simulink model "TST_CrCtl_ShOff"  (R2016b)
settings: Solver=FixedStepDiscrete  StartTime=0.0  StopTime=simTime  FixedStep=sampleTime  RelTol=1e-3
values from neighbouring files (symbols this model uses):
  testCase = 1    [initTST_CrCtl_ShOff_001.m]    (also in initTST_CrCtl_ShOff_002.m = 2; initTST_CrCtl_ShOff_003.m = 3)
libraries: simulink x31, UnitTest_Lib x15
(part 2 of 2)

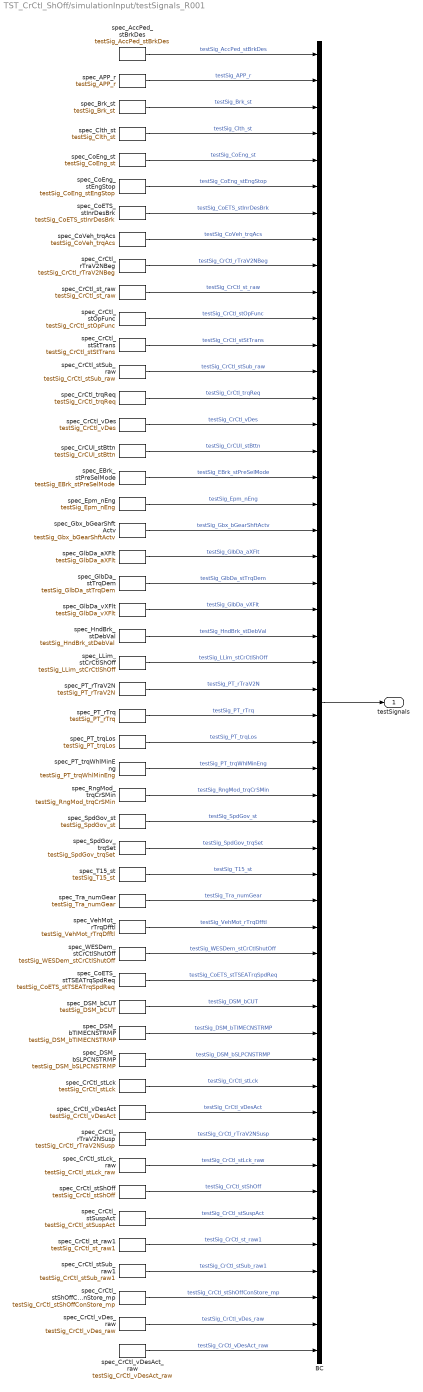
== system TST_CrCtl_ShOff/simulationInput/testSignals_R001 ==
  BC : BusCreator  Inputs=50
  spec_APP_r : FromWorkspace  VariableName=testSig_APP_r  Interpolate=off  OutputAfterFinalValue=Holding final value
  spec_AccPed_stBrkDes : FromWorkspace  VariableName=testSig_AccPed_stBrkDes  Interpolate=off  OutputAfterFinalValue=Holding final value
  spec_Brk_st : FromWorkspace  VariableName=testSig_Brk_st  Interpolate=off  OutputAfterFinalValue=Holding final value
  spec_Clth_st : FromWorkspace  VariableName=testSig_Clth_st  Interpolate=off  OutputAfterFinalValue=Holding final value
  spec_CoETS_stInrDesBrk : FromWorkspace  VariableName=testSig_CoETS_stInrDesBrk  Interpolate=off  OutputAfterFinalValue=Holding final value
  spec_CoETS_stTSEATrqSpdReq : FromWorkspace  VariableName=testSig_CoETS_stTSEATrqSpdReq  Interpolate=off  OutputAfterFinalValue=Holding final value
  spec_CoEng_st : FromWorkspace  VariableName=testSig_CoEng_st  Interpolate=off  OutputAfterFinalValue=Holding final value
  spec_CoEng_stEngStop : FromWorkspace  VariableName=testSig_CoEng_stEngStop  Interpolate=off  OutputAfterFinalValue=Holding final value
  spec_CoVeh_trqAcs : FromWorkspace  VariableName=testSig_CoVeh_trqAcs  Interpolate=off  OutputAfterFinalValue=Holding final value
  spec_CrCUI_stBttn : FromWorkspace  VariableName=testSig_CrCUI_stBttn  Interpolate=off  OutputAfterFinalValue=Holding final value
  spec_CrCtl_rTraV2NBeg : FromWorkspace  VariableName=testSig_CrCtl_rTraV2NBeg  Interpolate=off  OutputAfterFinalValue=Holding final value
  spec_CrCtl_rTraV2NSusp : FromWorkspace  VariableName=testSig_CrCtl_rTraV2NSusp  Interpolate=off  OutputAfterFinalValue=Holding final value
  spec_CrCtl_stLck : FromWorkspace  VariableName=testSig_CrCtl_stLck  Interpolate=off  OutputAfterFinalValue=Holding final value
  spec_CrCtl_stLck_raw : FromWorkspace  VariableName=testSig_CrCtl_stLck_raw  Interpolate=off  OutputAfterFinalValue=Holding final value
  spec_CrCtl_stOpFunc : FromWorkspace  VariableName=testSig_CrCtl_stOpFunc  Interpolate=off  OutputAfterFinalValue=Holding final value
  spec_CrCtl_stShOff : FromWorkspace  VariableName=testSig_CrCtl_stShOff  Interpolate=off  OutputAfterFinalValue=Holding final value
  spec_CrCtl_stShOffConStore_mp : FromWorkspace  VariableName=testSig_CrCtl_stShOffConStore_mp  Interpolate=off  OutputAfterFinalValue=Holding final value
  spec_CrCtl_stStTrans : FromWorkspace  VariableName=testSig_CrCtl_stStTrans  Interpolate=off  OutputAfterFinalValue=Holding final value
  spec_CrCtl_stSub_raw : FromWorkspace  VariableName=testSig_CrCtl_stSub_raw  Interpolate=off  OutputAfterFinalValue=Holding final value
  spec_CrCtl_stSub_raw1 : FromWorkspace  VariableName=testSig_CrCtl_stSub_raw1  Interpolate=off  OutputAfterFinalValue=Holding final value
  spec_CrCtl_stSuspAct : FromWorkspace  VariableName=testSig_CrCtl_stSuspAct  Interpolate=off  OutputAfterFinalValue=Holding final value
  spec_CrCtl_st_raw : FromWorkspace  VariableName=testSig_CrCtl_st_raw  Interpolate=off  OutputAfterFinalValue=Holding final value
  spec_CrCtl_st_raw1 : FromWorkspace  VariableName=testSig_CrCtl_st_raw1  Interpolate=off  OutputAfterFinalValue=Holding final value
  spec_CrCtl_trqReq : FromWorkspace  VariableName=testSig_CrCtl_trqReq  Interpolate=off  OutputAfterFinalValue=Holding final value
  spec_CrCtl_vDes : FromWorkspace  VariableName=testSig_CrCtl_vDes  Interpolate=off  OutputAfterFinalValue=Holding final value
  spec_CrCtl_vDesAct : FromWorkspace  VariableName=testSig_CrCtl_vDesAct  Interpolate=off  OutputAfterFinalValue=Holding final value
  spec_CrCtl_vDesAct_raw : FromWorkspace  VariableName=testSig_CrCtl_vDesAct_raw  Interpolate=off  OutputAfterFinalValue=Holding final value
  spec_CrCtl_vDes_raw : FromWorkspace  VariableName=testSig_CrCtl_vDes_raw  Interpolate=off  OutputAfterFinalValue=Holding final value
  spec_DSM_bCUT : FromWorkspace  VariableName=testSig_DSM_bCUT  Interpolate=off  OutputAfterFinalValue=Holding final value
  spec_DSM_bSLPCNSTRMP : FromWorkspace  VariableName=testSig_DSM_bSLPCNSTRMP  Interpolate=off  OutputAfterFinalValue=Holding final value
  spec_DSM_bTIMECNSTRMP : FromWorkspace  VariableName=testSig_DSM_bTIMECNSTRMP  Interpolate=off  OutputAfterFinalValue=Holding final value
  spec_EBrk_stPreSelMode : FromWorkspace  VariableName=testSig_EBrk_stPreSelMode  Interpolate=off  OutputAfterFinalValue=Holding final value
  spec_Epm_nEng : FromWorkspace  VariableName=testSig_Epm_nEng  Interpolate=off  OutputAfterFinalValue=Holding final value
  spec_Gbx_bGearShftActv : FromWorkspace  VariableName=testSig_Gbx_bGearShftActv  Interpolate=off  OutputAfterFinalValue=Holding final value
  spec_GlbDa_aXFlt : FromWorkspace  VariableName=testSig_GlbDa_aXFlt  Interpolate=off  OutputAfterFinalValue=Holding final value
  spec_GlbDa_stTrqDem : FromWorkspace  VariableName=testSig_GlbDa_stTrqDem  Interpolate=off  OutputAfterFinalValue=Holding final value
  spec_GlbDa_vXFlt : FromWorkspace  VariableName=testSig_GlbDa_vXFlt  Interpolate=off  OutputAfterFinalValue=Holding final value
  spec_HndBrk_stDebVal : FromWorkspace  VariableName=testSig_HndBrk_stDebVal  Interpolate=off  OutputAfterFinalValue=Holding final value
  spec_LLim_stCrCtlShOff : FromWorkspace  VariableName=testSig_LLim_stCrCtlShOff  Interpolate=off  OutputAfterFinalValue=Holding final value
  spec_PT_rTraV2N : FromWorkspace  VariableName=testSig_PT_rTraV2N  Interpolate=off  OutputAfterFinalValue=Holding final value
  spec_PT_rTrq : FromWorkspace  VariableName=testSig_PT_rTrq  Interpolate=off  OutputAfterFinalValue=Holding final value
  spec_PT_trqLos : FromWorkspace  VariableName=testSig_PT_trqLos  Interpolate=off  OutputAfterFinalValue=Holding final value
  spec_PT_trqWhlMinEng : FromWorkspace  VariableName=testSig_PT_trqWhlMinEng  Interpolate=off  OutputAfterFinalValue=Holding final value
  spec_RngMod_trqCrSMin : FromWorkspace  VariableName=testSig_RngMod_trqCrSMin  Interpolate=off  OutputAfterFinalValue=Holding final value
  spec_SpdGov_st : FromWorkspace  VariableName=testSig_SpdGov_st  Interpolate=off  OutputAfterFinalValue=Holding final value
  spec_SpdGov_trqSet : FromWorkspace  VariableName=testSig_SpdGov_trqSet  Interpolate=off  OutputAfterFinalValue=Holding final value
  spec_T15_st : FromWorkspace  VariableName=testSig_T15_st  Interpolate=off  OutputAfterFinalValue=Holding final value
  spec_Tra_numGear : FromWorkspace  VariableName=testSig_Tra_numGear  Interpolate=off  OutputAfterFinalValue=Holding final value
  spec_VehMot_rTrqDfftl : FromWorkspace  VariableName=testSig_VehMot_rTrqDfftl  Interpolate=off  OutputAfterFinalValue=Holding final value
  spec_WESDem_stCrCtlShutOff : FromWorkspace  VariableName=testSig_WESDem_stCrCtlShutOff  Interpolate=off  OutputAfterFinalValue=Holding final value
  testSignals : Outport
  wires:
  BC/1 -> testSignals/1
  spec_AccPed_stBrkDes/1 -> BC/1  "testSig_AccPed_stBrkDes"
  spec_APP_r/1 -> BC/2  "testSig_APP_r"
  spec_Brk_st/1 -> BC/3  "testSig_Brk_st"
  spec_Clth_st/1 -> BC/4  "testSig_Clth_st"
  spec_CoEng_st/1 -> BC/5  "testSig_CoEng_st"
  spec_CoEng_stEngStop/1 -> BC/6  "testSig_CoEng_stEngStop"
  spec_CoETS_stInrDesBrk/1 -> BC/7  "testSig_CoETS_stInrDesBrk"
  spec_CoVeh_trqAcs/1 -> BC/8  "testSig_CoVeh_trqAcs"
  spec_CrCtl_rTraV2NBeg/1 -> BC/9  "testSig_CrCtl_rTraV2NBeg"
  spec_CrCtl_st_raw/1 -> BC/10  "testSig_CrCtl_st_raw"
  spec_CrCtl_stOpFunc/1 -> BC/11  "testSig_CrCtl_stOpFunc"
  spec_CrCtl_stStTrans/1 -> BC/12  "testSig_CrCtl_stStTrans"
  spec_CrCtl_stSub_raw/1 -> BC/13  "testSig_CrCtl_stSub_raw"
  spec_CrCtl_trqReq/1 -> BC/14  "testSig_CrCtl_trqReq"
  spec_CrCtl_vDes/1 -> BC/15  "testSig_CrCtl_vDes"
  spec_CrCUI_stBttn/1 -> BC/16  "testSig_CrCUI_stBttn"
  spec_EBrk_stPreSelMode/1 -> BC/17  "testSig_EBrk_stPreSelMode"
  spec_Epm_nEng/1 -> BC/18  "testSig_Epm_nEng"
  spec_Gbx_bGearShftActv/1 -> BC/19  "testSig_Gbx_bGearShftActv"
  spec_GlbDa_aXFlt/1 -> BC/20  "testSig_GlbDa_aXFlt"
  spec_GlbDa_stTrqDem/1 -> BC/21  "testSig_GlbDa_stTrqDem"
  spec_GlbDa_vXFlt/1 -> BC/22  "testSig_GlbDa_vXFlt"
  spec_HndBrk_stDebVal/1 -> BC/23  "testSig_HndBrk_stDebVal"
  spec_LLim_stCrCtlShOff/1 -> BC/24  "testSig_LLim_stCrCtlShOff"
  spec_PT_rTraV2N/1 -> BC/25  "testSig_PT_rTraV2N"
  spec_PT_rTrq/1 -> BC/26  "testSig_PT_rTrq"
  spec_PT_trqLos/1 -> BC/27  "testSig_PT_trqLos"
  spec_PT_trqWhlMinEng/1 -> BC/28  "testSig_PT_trqWhlMinEng"
  spec_RngMod_trqCrSMin/1 -> BC/29  "testSig_RngMod_trqCrSMin"
  spec_SpdGov_st/1 -> BC/30  "testSig_SpdGov_st"
  spec_SpdGov_trqSet/1 -> BC/31  "testSig_SpdGov_trqSet"
  spec_T15_st/1 -> BC/32  "testSig_T15_st"
  spec_Tra_numGear/1 -> BC/33  "testSig_Tra_numGear"
  spec_VehMot_rTrqDfftl/1 -> BC/34  "testSig_VehMot_rTrqDfftl"
  spec_WESDem_stCrCtlShutOff/1 -> BC/35  "testSig_WESDem_stCrCtlShutOff"
  spec_CoETS_stTSEATrqSpdReq/1 -> BC/36  "testSig_CoETS_stTSEATrqSpdReq"
  spec_DSM_bCUT/1 -> BC/37  "testSig_DSM_bCUT"
  spec_DSM_bTIMECNSTRMP/1 -> BC/38  "testSig_DSM_bTIMECNSTRMP"
  spec_DSM_bSLPCNSTRMP/1 -> BC/39  "testSig_DSM_bSLPCNSTRMP"
  spec_CrCtl_stLck/1 -> BC/40  "testSig_CrCtl_stLck"
  spec_CrCtl_vDesAct/1 -> BC/41  "testSig_CrCtl_vDesAct"
  spec_CrCtl_rTraV2NSusp/1 -> BC/42  "testSig_CrCtl_rTraV2NSusp"
  spec_CrCtl_stLck_raw/1 -> BC/43  "testSig_CrCtl_stLck_raw"
  spec_CrCtl_stShOff/1 -> BC/44  "testSig_CrCtl_stShOff"
  spec_CrCtl_stSuspAct/1 -> BC/45  "testSig_CrCtl_stSuspAct"
  spec_CrCtl_st_raw1/1 -> BC/46  "testSig_CrCtl_st_raw1"
  spec_CrCtl_stSub_raw1/1 -> BC/47  "testSig_CrCtl_stSub_raw1"
  spec_CrCtl_stShOffConStore_mp/1 -> BC/48  "testSig_CrCtl_stShOffConStore_mp"
  spec_CrCtl_vDes_raw/1 -> BC/49  "testSig_CrCtl_vDes_raw"
  spec_CrCtl_vDesAct_raw/1 -> BC/50  "testSig_CrCtl_vDesAct_raw"

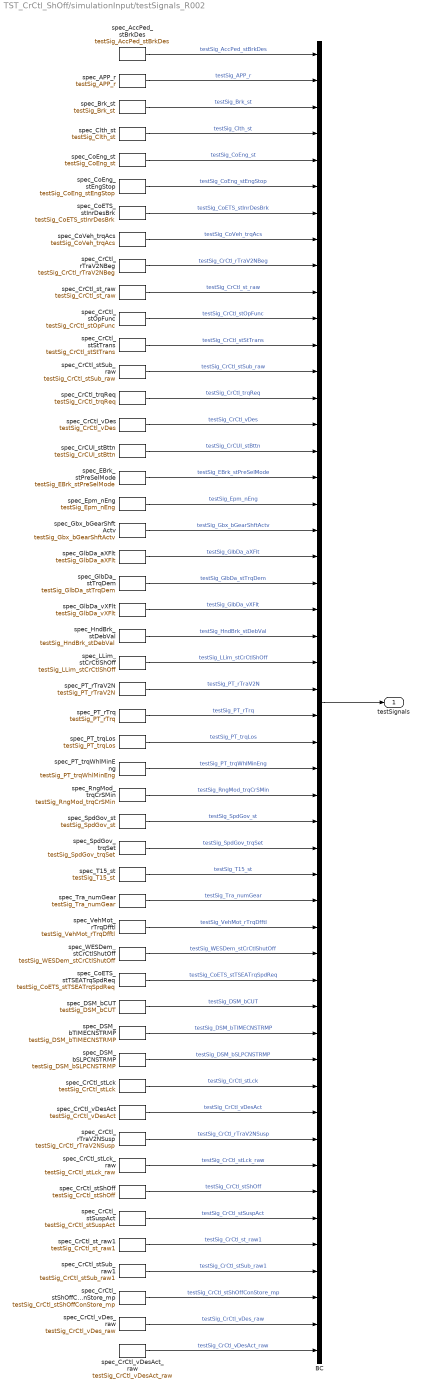
== system TST_CrCtl_ShOff/simulationInput/testSignals_R002 ==
  BC : BusCreator  Inputs=50
  spec_APP_r : FromWorkspace  VariableName=testSig_APP_r  Interpolate=off  OutputAfterFinalValue=Holding final value
  spec_AccPed_stBrkDes : FromWorkspace  VariableName=testSig_AccPed_stBrkDes  Interpolate=off  OutputAfterFinalValue=Holding final value
  spec_Brk_st : FromWorkspace  VariableName=testSig_Brk_st  Interpolate=off  OutputAfterFinalValue=Holding final value
  spec_Clth_st : FromWorkspace  VariableName=testSig_Clth_st  Interpolate=off  OutputAfterFinalValue=Holding final value
  spec_CoETS_stInrDesBrk : FromWorkspace  VariableName=testSig_CoETS_stInrDesBrk  Interpolate=off  OutputAfterFinalValue=Holding final value
  spec_CoETS_stTSEATrqSpdReq : FromWorkspace  VariableName=testSig_CoETS_stTSEATrqSpdReq  Interpolate=off  OutputAfterFinalValue=Holding final value
  spec_CoEng_st : FromWorkspace  VariableName=testSig_CoEng_st  Interpolate=off  OutputAfterFinalValue=Holding final value
  spec_CoEng_stEngStop : FromWorkspace  VariableName=testSig_CoEng_stEngStop  Interpolate=off  OutputAfterFinalValue=Holding final value
  spec_CoVeh_trqAcs : FromWorkspace  VariableName=testSig_CoVeh_trqAcs  Interpolate=off  OutputAfterFinalValue=Holding final value
  spec_CrCUI_stBttn : FromWorkspace  VariableName=testSig_CrCUI_stBttn  Interpolate=off  OutputAfterFinalValue=Holding final value
  spec_CrCtl_rTraV2NBeg : FromWorkspace  VariableName=testSig_CrCtl_rTraV2NBeg  Interpolate=off  OutputAfterFinalValue=Holding final value
  spec_CrCtl_rTraV2NSusp : FromWorkspace  VariableName=testSig_CrCtl_rTraV2NSusp  Interpolate=off  OutputAfterFinalValue=Holding final value
  spec_CrCtl_stLck : FromWorkspace  VariableName=testSig_CrCtl_stLck  Interpolate=off  OutputAfterFinalValue=Holding final value
  spec_CrCtl_stLck_raw : FromWorkspace  VariableName=testSig_CrCtl_stLck_raw  Interpolate=off  OutputAfterFinalValue=Holding final value
  spec_CrCtl_stOpFunc : FromWorkspace  VariableName=testSig_CrCtl_stOpFunc  Interpolate=off  OutputAfterFinalValue=Holding final value
  spec_CrCtl_stShOff : FromWorkspace  VariableName=testSig_CrCtl_stShOff  Interpolate=off  OutputAfterFinalValue=Holding final value
  spec_CrCtl_stShOffConStore_mp : FromWorkspace  VariableName=testSig_CrCtl_stShOffConStore_mp  Interpolate=off  OutputAfterFinalValue=Holding final value
  spec_CrCtl_stStTrans : FromWorkspace  VariableName=testSig_CrCtl_stStTrans  Interpolate=off  OutputAfterFinalValue=Holding final value
  spec_CrCtl_stSub_raw : FromWorkspace  VariableName=testSig_CrCtl_stSub_raw  Interpolate=off  OutputAfterFinalValue=Holding final value
  spec_CrCtl_stSub_raw1 : FromWorkspace  VariableName=testSig_CrCtl_stSub_raw1  Interpolate=off  OutputAfterFinalValue=Holding final value
  spec_CrCtl_stSuspAct : FromWorkspace  VariableName=testSig_CrCtl_stSuspAct  Interpolate=off  OutputAfterFinalValue=Holding final value
  spec_CrCtl_st_raw : FromWorkspace  VariableName=testSig_CrCtl_st_raw  Interpolate=off  OutputAfterFinalValue=Holding final value
  spec_CrCtl_st_raw1 : FromWorkspace  VariableName=testSig_CrCtl_st_raw1  Interpolate=off  OutputAfterFinalValue=Holding final value
  spec_CrCtl_trqReq : FromWorkspace  VariableName=testSig_CrCtl_trqReq  Interpolate=off  OutputAfterFinalValue=Holding final value
  spec_CrCtl_vDes : FromWorkspace  VariableName=testSig_CrCtl_vDes  Interpolate=off  OutputAfterFinalValue=Holding final value
  spec_CrCtl_vDesAct : FromWorkspace  VariableName=testSig_CrCtl_vDesAct  Interpolate=off  OutputAfterFinalValue=Holding final value
  spec_CrCtl_vDesAct_raw : FromWorkspace  VariableName=testSig_CrCtl_vDesAct_raw  Interpolate=off  OutputAfterFinalValue=Holding final value
  spec_CrCtl_vDes_raw : FromWorkspace  VariableName=testSig_CrCtl_vDes_raw  Interpolate=off  OutputAfterFinalValue=Holding final value
  spec_DSM_bCUT : FromWorkspace  VariableName=testSig_DSM_bCUT  Interpolate=off  OutputAfterFinalValue=Holding final value
  spec_DSM_bSLPCNSTRMP : FromWorkspace  VariableName=testSig_DSM_bSLPCNSTRMP  Interpolate=off  OutputAfterFinalValue=Holding final value
  spec_DSM_bTIMECNSTRMP : FromWorkspace  VariableName=testSig_DSM_bTIMECNSTRMP  Interpolate=off  OutputAfterFinalValue=Holding final value
  spec_EBrk_stPreSelMode : FromWorkspace  VariableName=testSig_EBrk_stPreSelMode  Interpolate=off  OutputAfterFinalValue=Holding final value
  spec_Epm_nEng : FromWorkspace  VariableName=testSig_Epm_nEng  Interpolate=off  OutputAfterFinalValue=Holding final value
  spec_Gbx_bGearShftActv : FromWorkspace  VariableName=testSig_Gbx_bGearShftActv  Interpolate=off  OutputAfterFinalValue=Holding final value
  spec_GlbDa_aXFlt : FromWorkspace  VariableName=testSig_GlbDa_aXFlt  Interpolate=off  OutputAfterFinalValue=Holding final value
  spec_GlbDa_stTrqDem : FromWorkspace  VariableName=testSig_GlbDa_stTrqDem  Interpolate=off  OutputAfterFinalValue=Holding final value
  spec_GlbDa_vXFlt : FromWorkspace  VariableName=testSig_GlbDa_vXFlt  Interpolate=off  OutputAfterFinalValue=Holding final value
  spec_HndBrk_stDebVal : FromWorkspace  VariableName=testSig_HndBrk_stDebVal  Interpolate=off  OutputAfterFinalValue=Holding final value
  spec_LLim_stCrCtlShOff : FromWorkspace  VariableName=testSig_LLim_stCrCtlShOff  Interpolate=off  OutputAfterFinalValue=Holding final value
  spec_PT_rTraV2N : FromWorkspace  VariableName=testSig_PT_rTraV2N  Interpolate=off  OutputAfterFinalValue=Holding final value
  spec_PT_rTrq : FromWorkspace  VariableName=testSig_PT_rTrq  Interpolate=off  OutputAfterFinalValue=Holding final value
  spec_PT_trqLos : FromWorkspace  VariableName=testSig_PT_trqLos  Interpolate=off  OutputAfterFinalValue=Holding final value
  spec_PT_trqWhlMinEng : FromWorkspace  VariableName=testSig_PT_trqWhlMinEng  Interpolate=off  OutputAfterFinalValue=Holding final value
  spec_RngMod_trqCrSMin : FromWorkspace  VariableName=testSig_RngMod_trqCrSMin  Interpolate=off  OutputAfterFinalValue=Holding final value
  spec_SpdGov_st : FromWorkspace  VariableName=testSig_SpdGov_st  Interpolate=off  OutputAfterFinalValue=Holding final value
  spec_SpdGov_trqSet : FromWorkspace  VariableName=testSig_SpdGov_trqSet  Interpolate=off  OutputAfterFinalValue=Holding final value
  spec_T15_st : FromWorkspace  VariableName=testSig_T15_st  Interpolate=off  OutputAfterFinalValue=Holding final value
  spec_Tra_numGear : FromWorkspace  VariableName=testSig_Tra_numGear  Interpolate=off  OutputAfterFinalValue=Holding final value
  spec_VehMot_rTrqDfftl : FromWorkspace  VariableName=testSig_VehMot_rTrqDfftl  Interpolate=off  OutputAfterFinalValue=Holding final value
  spec_WESDem_stCrCtlShutOff : FromWorkspace  VariableName=testSig_WESDem_stCrCtlShutOff  Interpolate=off  OutputAfterFinalValue=Holding final value
  testSignals : Outport
  wires:
  BC/1 -> testSignals/1
  spec_AccPed_stBrkDes/1 -> BC/1  "testSig_AccPed_stBrkDes"
  spec_APP_r/1 -> BC/2  "testSig_APP_r"
  spec_Brk_st/1 -> BC/3  "testSig_Brk_st"
  spec_Clth_st/1 -> BC/4  "testSig_Clth_st"
  spec_CoEng_st/1 -> BC/5  "testSig_CoEng_st"
  spec_CoEng_stEngStop/1 -> BC/6  "testSig_CoEng_stEngStop"
  spec_CoETS_stInrDesBrk/1 -> BC/7  "testSig_CoETS_stInrDesBrk"
  spec_CoVeh_trqAcs/1 -> BC/8  "testSig_CoVeh_trqAcs"
  spec_CrCtl_rTraV2NBeg/1 -> BC/9  "testSig_CrCtl_rTraV2NBeg"
  spec_CrCtl_st_raw/1 -> BC/10  "testSig_CrCtl_st_raw"
  spec_CrCtl_stOpFunc/1 -> BC/11  "testSig_CrCtl_stOpFunc"
  spec_CrCtl_stStTrans/1 -> BC/12  "testSig_CrCtl_stStTrans"
  spec_CrCtl_stSub_raw/1 -> BC/13  "testSig_CrCtl_stSub_raw"
  spec_CrCtl_trqReq/1 -> BC/14  "testSig_CrCtl_trqReq"
  spec_CrCtl_vDes/1 -> BC/15  "testSig_CrCtl_vDes"
  spec_CrCUI_stBttn/1 -> BC/16  "testSig_CrCUI_stBttn"
  spec_EBrk_stPreSelMode/1 -> BC/17  "testSig_EBrk_stPreSelMode"
  spec_Epm_nEng/1 -> BC/18  "testSig_Epm_nEng"
  spec_Gbx_bGearShftActv/1 -> BC/19  "testSig_Gbx_bGearShftActv"
  spec_GlbDa_aXFlt/1 -> BC/20  "testSig_GlbDa_aXFlt"
  spec_GlbDa_stTrqDem/1 -> BC/21  "testSig_GlbDa_stTrqDem"
  spec_GlbDa_vXFlt/1 -> BC/22  "testSig_GlbDa_vXFlt"
  spec_HndBrk_stDebVal/1 -> BC/23  "testSig_HndBrk_stDebVal"
  spec_LLim_stCrCtlShOff/1 -> BC/24  "testSig_LLim_stCrCtlShOff"
  spec_PT_rTraV2N/1 -> BC/25  "testSig_PT_rTraV2N"
  spec_PT_rTrq/1 -> BC/26  "testSig_PT_rTrq"
  spec_PT_trqLos/1 -> BC/27  "testSig_PT_trqLos"
  spec_PT_trqWhlMinEng/1 -> BC/28  "testSig_PT_trqWhlMinEng"
  spec_RngMod_trqCrSMin/1 -> BC/29  "testSig_RngMod_trqCrSMin"
  spec_SpdGov_st/1 -> BC/30  "testSig_SpdGov_st"
  spec_SpdGov_trqSet/1 -> BC/31  "testSig_SpdGov_trqSet"
  spec_T15_st/1 -> BC/32  "testSig_T15_st"
  spec_Tra_numGear/1 -> BC/33  "testSig_Tra_numGear"
  spec_VehMot_rTrqDfftl/1 -> BC/34  "testSig_VehMot_rTrqDfftl"
  spec_WESDem_stCrCtlShutOff/1 -> BC/35  "testSig_WESDem_stCrCtlShutOff"
  spec_CoETS_stTSEATrqSpdReq/1 -> BC/36  "testSig_CoETS_stTSEATrqSpdReq"
  spec_DSM_bCUT/1 -> BC/37  "testSig_DSM_bCUT"
  spec_DSM_bTIMECNSTRMP/1 -> BC/38  "testSig_DSM_bTIMECNSTRMP"
  spec_DSM_bSLPCNSTRMP/1 -> BC/39  "testSig_DSM_bSLPCNSTRMP"
  spec_CrCtl_stLck/1 -> BC/40  "testSig_CrCtl_stLck"
  spec_CrCtl_vDesAct/1 -> BC/41  "testSig_CrCtl_vDesAct"
  spec_CrCtl_rTraV2NSusp/1 -> BC/42  "testSig_CrCtl_rTraV2NSusp"
  spec_CrCtl_stLck_raw/1 -> BC/43  "testSig_CrCtl_stLck_raw"
  spec_CrCtl_stShOff/1 -> BC/44  "testSig_CrCtl_stShOff"
  spec_CrCtl_stSuspAct/1 -> BC/45  "testSig_CrCtl_stSuspAct"
  spec_CrCtl_st_raw1/1 -> BC/46  "testSig_CrCtl_st_raw1"
  spec_CrCtl_stSub_raw1/1 -> BC/47  "testSig_CrCtl_stSub_raw1"
  spec_CrCtl_stShOffConStore_mp/1 -> BC/48  "testSig_CrCtl_stShOffConStore_mp"
  spec_CrCtl_vDes_raw/1 -> BC/49  "testSig_CrCtl_vDes_raw"
  spec_CrCtl_vDesAct_raw/1 -> BC/50  "testSig_CrCtl_vDesAct_raw"

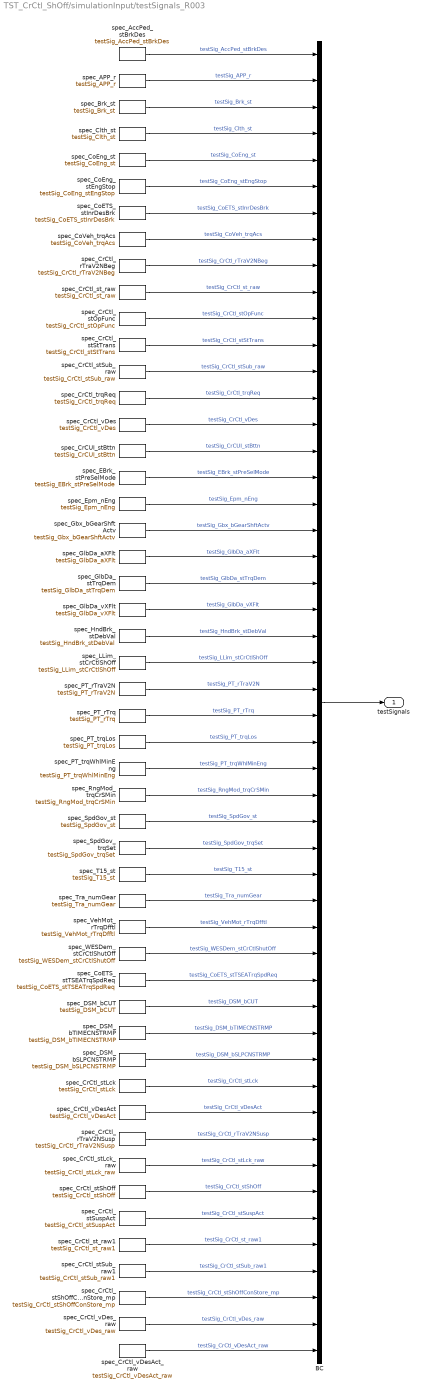
== system TST_CrCtl_ShOff/simulationInput/testSignals_R003 ==
  BC : BusCreator  Inputs=50
  spec_APP_r : FromWorkspace  VariableName=testSig_APP_r  Interpolate=off  OutputAfterFinalValue=Holding final value
  spec_AccPed_stBrkDes : FromWorkspace  VariableName=testSig_AccPed_stBrkDes  Interpolate=off  OutputAfterFinalValue=Holding final value
  spec_Brk_st : FromWorkspace  VariableName=testSig_Brk_st  Interpolate=off  OutputAfterFinalValue=Holding final value
  spec_Clth_st : FromWorkspace  VariableName=testSig_Clth_st  Interpolate=off  OutputAfterFinalValue=Holding final value
  spec_CoETS_stInrDesBrk : FromWorkspace  VariableName=testSig_CoETS_stInrDesBrk  Interpolate=off  OutputAfterFinalValue=Holding final value
  spec_CoETS_stTSEATrqSpdReq : FromWorkspace  VariableName=testSig_CoETS_stTSEATrqSpdReq  Interpolate=off  OutputAfterFinalValue=Holding final value
  spec_CoEng_st : FromWorkspace  VariableName=testSig_CoEng_st  Interpolate=off  OutputAfterFinalValue=Holding final value
  spec_CoEng_stEngStop : FromWorkspace  VariableName=testSig_CoEng_stEngStop  Interpolate=off  OutputAfterFinalValue=Holding final value
  spec_CoVeh_trqAcs : FromWorkspace  VariableName=testSig_CoVeh_trqAcs  Interpolate=off  OutputAfterFinalValue=Holding final value
  spec_CrCUI_stBttn : FromWorkspace  VariableName=testSig_CrCUI_stBttn  Interpolate=off  OutputAfterFinalValue=Holding final value
  spec_CrCtl_rTraV2NBeg : FromWorkspace  VariableName=testSig_CrCtl_rTraV2NBeg  Interpolate=off  OutputAfterFinalValue=Holding final value
  spec_CrCtl_rTraV2NSusp : FromWorkspace  VariableName=testSig_CrCtl_rTraV2NSusp  Interpolate=off  OutputAfterFinalValue=Holding final value
  spec_CrCtl_stLck : FromWorkspace  VariableName=testSig_CrCtl_stLck  Interpolate=off  OutputAfterFinalValue=Holding final value
  spec_CrCtl_stLck_raw : FromWorkspace  VariableName=testSig_CrCtl_stLck_raw  Interpolate=off  OutputAfterFinalValue=Holding final value
  spec_CrCtl_stOpFunc : FromWorkspace  VariableName=testSig_CrCtl_stOpFunc  Interpolate=off  OutputAfterFinalValue=Holding final value
  spec_CrCtl_stShOff : FromWorkspace  VariableName=testSig_CrCtl_stShOff  Interpolate=off  OutputAfterFinalValue=Holding final value
  spec_CrCtl_stShOffConStore_mp : FromWorkspace  VariableName=testSig_CrCtl_stShOffConStore_mp  Interpolate=off  OutputAfterFinalValue=Holding final value
  spec_CrCtl_stStTrans : FromWorkspace  VariableName=testSig_CrCtl_stStTrans  Interpolate=off  OutputAfterFinalValue=Holding final value
  spec_CrCtl_stSub_raw : FromWorkspace  VariableName=testSig_CrCtl_stSub_raw  Interpolate=off  OutputAfterFinalValue=Holding final value
  spec_CrCtl_stSub_raw1 : FromWorkspace  VariableName=testSig_CrCtl_stSub_raw1  Interpolate=off  OutputAfterFinalValue=Holding final value
  spec_CrCtl_stSuspAct : FromWorkspace  VariableName=testSig_CrCtl_stSuspAct  Interpolate=off  OutputAfterFinalValue=Holding final value
  spec_CrCtl_st_raw : FromWorkspace  VariableName=testSig_CrCtl_st_raw  Interpolate=off  OutputAfterFinalValue=Holding final value
  spec_CrCtl_st_raw1 : FromWorkspace  VariableName=testSig_CrCtl_st_raw1  Interpolate=off  OutputAfterFinalValue=Holding final value
  spec_CrCtl_trqReq : FromWorkspace  VariableName=testSig_CrCtl_trqReq  Interpolate=off  OutputAfterFinalValue=Holding final value
  spec_CrCtl_vDes : FromWorkspace  VariableName=testSig_CrCtl_vDes  Interpolate=off  OutputAfterFinalValue=Holding final value
  spec_CrCtl_vDesAct : FromWorkspace  VariableName=testSig_CrCtl_vDesAct  Interpolate=off  OutputAfterFinalValue=Holding final value
  spec_CrCtl_vDesAct_raw : FromWorkspace  VariableName=testSig_CrCtl_vDesAct_raw  Interpolate=off  OutputAfterFinalValue=Holding final value
  spec_CrCtl_vDes_raw : FromWorkspace  VariableName=testSig_CrCtl_vDes_raw  Interpolate=off  OutputAfterFinalValue=Holding final value
  spec_DSM_bCUT : FromWorkspace  VariableName=testSig_DSM_bCUT  Interpolate=off  OutputAfterFinalValue=Holding final value
  spec_DSM_bSLPCNSTRMP : FromWorkspace  VariableName=testSig_DSM_bSLPCNSTRMP  Interpolate=off  OutputAfterFinalValue=Holding final value
  spec_DSM_bTIMECNSTRMP : FromWorkspace  VariableName=testSig_DSM_bTIMECNSTRMP  Interpolate=off  OutputAfterFinalValue=Holding final value
  spec_EBrk_stPreSelMode : FromWorkspace  VariableName=testSig_EBrk_stPreSelMode  Interpolate=off  OutputAfterFinalValue=Holding final value
  spec_Epm_nEng : FromWorkspace  VariableName=testSig_Epm_nEng  Interpolate=off  OutputAfterFinalValue=Holding final value
  spec_Gbx_bGearShftActv : FromWorkspace  VariableName=testSig_Gbx_bGearShftActv  Interpolate=off  OutputAfterFinalValue=Holding final value
  spec_GlbDa_aXFlt : FromWorkspace  VariableName=testSig_GlbDa_aXFlt  Interpolate=off  OutputAfterFinalValue=Holding final value
  spec_GlbDa_stTrqDem : FromWorkspace  VariableName=testSig_GlbDa_stTrqDem  Interpolate=off  OutputAfterFinalValue=Holding final value
  spec_GlbDa_vXFlt : FromWorkspace  VariableName=testSig_GlbDa_vXFlt  Interpolate=off  OutputAfterFinalValue=Holding final value
  spec_HndBrk_stDebVal : FromWorkspace  VariableName=testSig_HndBrk_stDebVal  Interpolate=off  OutputAfterFinalValue=Holding final value
  spec_LLim_stCrCtlShOff : FromWorkspace  VariableName=testSig_LLim_stCrCtlShOff  Interpolate=off  OutputAfterFinalValue=Holding final value
  spec_PT_rTraV2N : FromWorkspace  VariableName=testSig_PT_rTraV2N  Interpolate=off  OutputAfterFinalValue=Holding final value
  spec_PT_rTrq : FromWorkspace  VariableName=testSig_PT_rTrq  Interpolate=off  OutputAfterFinalValue=Holding final value
  spec_PT_trqLos : FromWorkspace  VariableName=testSig_PT_trqLos  Interpolate=off  OutputAfterFinalValue=Holding final value
  spec_PT_trqWhlMinEng : FromWorkspace  VariableName=testSig_PT_trqWhlMinEng  Interpolate=off  OutputAfterFinalValue=Holding final value
  spec_RngMod_trqCrSMin : FromWorkspace  VariableName=testSig_RngMod_trqCrSMin  Interpolate=off  OutputAfterFinalValue=Holding final value
  spec_SpdGov_st : FromWorkspace  VariableName=testSig_SpdGov_st  Interpolate=off  OutputAfterFinalValue=Holding final value
  spec_SpdGov_trqSet : FromWorkspace  VariableName=testSig_SpdGov_trqSet  Interpolate=off  OutputAfterFinalValue=Holding final value
  spec_T15_st : FromWorkspace  VariableName=testSig_T15_st  Interpolate=off  OutputAfterFinalValue=Holding final value
  spec_Tra_numGear : FromWorkspace  VariableName=testSig_Tra_numGear  Interpolate=off  OutputAfterFinalValue=Holding final value
  spec_VehMot_rTrqDfftl : FromWorkspace  VariableName=testSig_VehMot_rTrqDfftl  Interpolate=off  OutputAfterFinalValue=Holding final value
  spec_WESDem_stCrCtlShutOff : FromWorkspace  VariableName=testSig_WESDem_stCrCtlShutOff  Interpolate=off  OutputAfterFinalValue=Holding final value
  testSignals : Outport
  wires:
  BC/1 -> testSignals/1
  spec_AccPed_stBrkDes/1 -> BC/1  "testSig_AccPed_stBrkDes"
  spec_APP_r/1 -> BC/2  "testSig_APP_r"
  spec_Brk_st/1 -> BC/3  "testSig_Brk_st"
  spec_Clth_st/1 -> BC/4  "testSig_Clth_st"
  spec_CoEng_st/1 -> BC/5  "testSig_CoEng_st"
  spec_CoEng_stEngStop/1 -> BC/6  "testSig_CoEng_stEngStop"
  spec_CoETS_stInrDesBrk/1 -> BC/7  "testSig_CoETS_stInrDesBrk"
  spec_CoVeh_trqAcs/1 -> BC/8  "testSig_CoVeh_trqAcs"
  spec_CrCtl_rTraV2NBeg/1 -> BC/9  "testSig_CrCtl_rTraV2NBeg"
  spec_CrCtl_st_raw/1 -> BC/10  "testSig_CrCtl_st_raw"
  spec_CrCtl_stOpFunc/1 -> BC/11  "testSig_CrCtl_stOpFunc"
  spec_CrCtl_stStTrans/1 -> BC/12  "testSig_CrCtl_stStTrans"
  spec_CrCtl_stSub_raw/1 -> BC/13  "testSig_CrCtl_stSub_raw"
  spec_CrCtl_trqReq/1 -> BC/14  "testSig_CrCtl_trqReq"
  spec_CrCtl_vDes/1 -> BC/15  "testSig_CrCtl_vDes"
  spec_CrCUI_stBttn/1 -> BC/16  "testSig_CrCUI_stBttn"
  spec_EBrk_stPreSelMode/1 -> BC/17  "testSig_EBrk_stPreSelMode"
  spec_Epm_nEng/1 -> BC/18  "testSig_Epm_nEng"
  spec_Gbx_bGearShftActv/1 -> BC/19  "testSig_Gbx_bGearShftActv"
  spec_GlbDa_aXFlt/1 -> BC/20  "testSig_GlbDa_aXFlt"
  spec_GlbDa_stTrqDem/1 -> BC/21  "testSig_GlbDa_stTrqDem"
  spec_GlbDa_vXFlt/1 -> BC/22  "testSig_GlbDa_vXFlt"
  spec_HndBrk_stDebVal/1 -> BC/23  "testSig_HndBrk_stDebVal"
  spec_LLim_stCrCtlShOff/1 -> BC/24  "testSig_LLim_stCrCtlShOff"
  spec_PT_rTraV2N/1 -> BC/25  "testSig_PT_rTraV2N"
  spec_PT_rTrq/1 -> BC/26  "testSig_PT_rTrq"
  spec_PT_trqLos/1 -> BC/27  "testSig_PT_trqLos"
  spec_PT_trqWhlMinEng/1 -> BC/28  "testSig_PT_trqWhlMinEng"
  spec_RngMod_trqCrSMin/1 -> BC/29  "testSig_RngMod_trqCrSMin"
  spec_SpdGov_st/1 -> BC/30  "testSig_SpdGov_st"
  spec_SpdGov_trqSet/1 -> BC/31  "testSig_SpdGov_trqSet"
  spec_T15_st/1 -> BC/32  "testSig_T15_st"
  spec_Tra_numGear/1 -> BC/33  "testSig_Tra_numGear"
  spec_VehMot_rTrqDfftl/1 -> BC/34  "testSig_VehMot_rTrqDfftl"
  spec_WESDem_stCrCtlShutOff/1 -> BC/35  "testSig_WESDem_stCrCtlShutOff"
  spec_CoETS_stTSEATrqSpdReq/1 -> BC/36  "testSig_CoETS_stTSEATrqSpdReq"
  spec_DSM_bCUT/1 -> BC/37  "testSig_DSM_bCUT"
  spec_DSM_bTIMECNSTRMP/1 -> BC/38  "testSig_DSM_bTIMECNSTRMP"
  spec_DSM_bSLPCNSTRMP/1 -> BC/39  "testSig_DSM_bSLPCNSTRMP"
  spec_CrCtl_stLck/1 -> BC/40  "testSig_CrCtl_stLck"
  spec_CrCtl_vDesAct/1 -> BC/41  "testSig_CrCtl_vDesAct"
  spec_CrCtl_rTraV2NSusp/1 -> BC/42  "testSig_CrCtl_rTraV2NSusp"
  spec_CrCtl_stLck_raw/1 -> BC/43  "testSig_CrCtl_stLck_raw"
  spec_CrCtl_stShOff/1 -> BC/44  "testSig_CrCtl_stShOff"
  spec_CrCtl_stSuspAct/1 -> BC/45  "testSig_CrCtl_stSuspAct"
  spec_CrCtl_st_raw1/1 -> BC/46  "testSig_CrCtl_st_raw1"
  spec_CrCtl_stSub_raw1/1 -> BC/47  "testSig_CrCtl_stSub_raw1"
  spec_CrCtl_stShOffConStore_mp/1 -> BC/48  "testSig_CrCtl_stShOffConStore_mp"
  spec_CrCtl_vDes_raw/1 -> BC/49  "testSig_CrCtl_vDes_raw"
  spec_CrCtl_vDesAct_raw/1 -> BC/50  "testSig_CrCtl_vDesAct_raw"

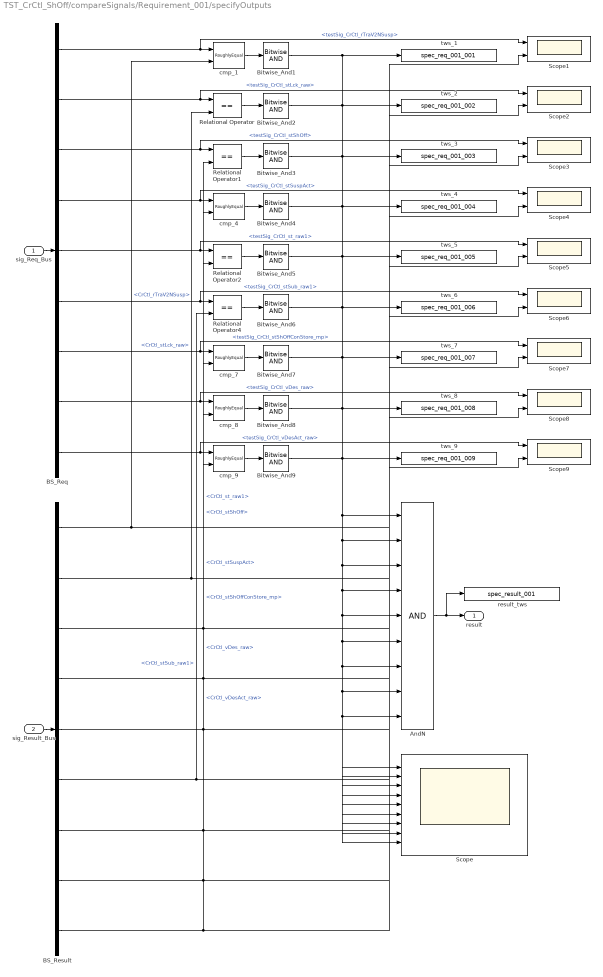
== system TST_CrCtl_ShOff/compareSignals/Requirement_001/specifyOutputs ==
  sig_Req_Bus : Inport
  sig_Result_Bus : Inport  Port=2
  AndN : Logic  Inputs=9
  BS_Req : BusSelector  OutputSignals=testSig_CrCtl_rTraV2NSusp,testSig_CrCtl_stLck_raw,testSig_CrCtl_stShOff,testSig_CrCtl_stSuspAct,testSig_CrCtl_st_raw1,testSig_CrCtl_stSub_raw1,testSig_CrCtl_stShOffConStore_mp,testSig_CrCtl_vDes_raw,testSig_CrCtl_vDesAct_raw
  BS_Result : BusSelector  OutputSignals=CrCtl_rTraV2NSusp,CrCtl_stLck_raw,CrCtl_stShOff,CrCtl_stSuspAct,CrCtl_st_raw1,CrCtl_stSub_raw1,CrCtl_stShOffConStore_mp,CrCtl_vDes_raw,CrCtl_vDesAct_raw
  Bitwise_And{1..9} (9 alike) : simulink/Logic and Bit Operations/Bitwise Operator  logicop=AND  UseBitMask=off  BitMask=bin2dec('11011001')  BitMaskRealWorld=Stored Integer
  Relational Operator{,1..2,4} (4 alike) : RelationalOperator  Operator===  OutDataTypeStr=boolean  RndMeth=Simplest
  Scope : Scope  NumInputPorts=9
  Scope{1..9} (9 alike) : Scope  NumInputPorts=2
  cmp_{1,4,7..9} (5 alike) : UnitTest_Lib/RoughlyEqual  slope=0.1
  result_tws : ToWorkspace  VariableName=spec_result_001
  tws_1 : ToWorkspace  VariableName=spec_req_001_001
  tws_2 : ToWorkspace  VariableName=spec_req_001_002
  tws_3 : ToWorkspace  VariableName=spec_req_001_003
  tws_4 : ToWorkspace  VariableName=spec_req_001_004
  tws_5 : ToWorkspace  VariableName=spec_req_001_005
  tws_6 : ToWorkspace  VariableName=spec_req_001_006
  tws_7 : ToWorkspace  VariableName=spec_req_001_007
  tws_8 : ToWorkspace  VariableName=spec_req_001_008
  tws_9 : ToWorkspace  VariableName=spec_req_001_009
  result : Outport
  wires:
  sig_Req_Bus/1 -> BS_Req/1
  sig_Result_Bus/1 -> BS_Result/1
  AndN/1 -> result/1, result_tws/1
  BS_Req/1 -> cmp_1/1, Scope1/1  "<testSig_CrCtl_rTraV2NSusp>"
  BS_Result/1 -> cmp_1/2, Scope1/2  "<CrCtl_rTraV2NSusp>"
  cmp_1/1 -> Bitwise_And1/1
  Bitwise_And1/1 -> AndN/1, Scope/1, tws_1/1
  BS_Req/2 -> Relational Operator/1, Scope2/1  "<testSig_CrCtl_stLck_raw>"
  BS_Result/2 -> Scope2/2, Relational Operator/2  "<CrCtl_stLck_raw>"
  Relational Operator/1 -> Bitwise_And2/1
  Bitwise_And2/1 -> AndN/2, Scope/2, tws_2/1
  BS_Req/3 -> Relational Operator1/1, Scope3/1  "<testSig_CrCtl_stShOff>"
  BS_Result/3 -> Relational Operator1/2, Scope3/2  "<CrCtl_stShOff>"
  Relational Operator1/1 -> Bitwise_And3/1
  Bitwise_And3/1 -> AndN/3, Scope/3, tws_3/1
  BS_Req/4 -> cmp_4/1, Scope4/1  "<testSig_CrCtl_stSuspAct>"
  BS_Result/4 -> cmp_4/2, Scope4/2  "<CrCtl_stSuspAct>"
  cmp_4/1 -> Bitwise_And4/1
  Bitwise_And4/1 -> AndN/4, Scope/4, tws_4/1
  BS_Req/5 -> Relational Operator2/1, Scope5/1  "<testSig_CrCtl_st_raw1>"
  BS_Result/5 -> Relational Operator2/2, Scope5/2  "<CrCtl_st_raw1>"
  Relational Operator2/1 -> Bitwise_And5/1
  Bitwise_And5/1 -> AndN/5, Scope/5, tws_5/1
  BS_Req/6 -> Relational Operator4/1, Scope6/1  "<testSig_CrCtl_stSub_raw1>"
  BS_Result/6 -> Scope6/2, Relational Operator4/2  "<CrCtl_stSub_raw1>"
  Relational Operator4/1 -> Bitwise_And6/1
  Bitwise_And6/1 -> AndN/6, Scope/6, tws_6/1
  BS_Req/7 -> cmp_7/1, Scope7/1  "<testSig_CrCtl_stShOffConStore_mp>"
  BS_Result/7 -> cmp_7/2, Scope7/2  "<CrCtl_stShOffConStore_mp>"
  cmp_7/1 -> Bitwise_And7/1
  Bitwise_And7/1 -> AndN/7, Scope/7, tws_7/1
  BS_Req/8 -> cmp_8/1, Scope8/1  "<testSig_CrCtl_vDes_raw>"
  BS_Result/8 -> cmp_8/2, Scope8/2  "<CrCtl_vDes_raw>"
  cmp_8/1 -> Bitwise_And8/1
  Bitwise_And8/1 -> AndN/8, Scope/8, tws_8/1
  BS_Req/9 -> cmp_9/1, Scope9/1  "<testSig_CrCtl_vDesAct_raw>"
  BS_Result/9 -> cmp_9/2, Scope9/2  "<CrCtl_vDesAct_raw>"
  cmp_9/1 -> Bitwise_And9/1
  Bitwise_And9/1 -> AndN/9, Scope/9, tws_9/1

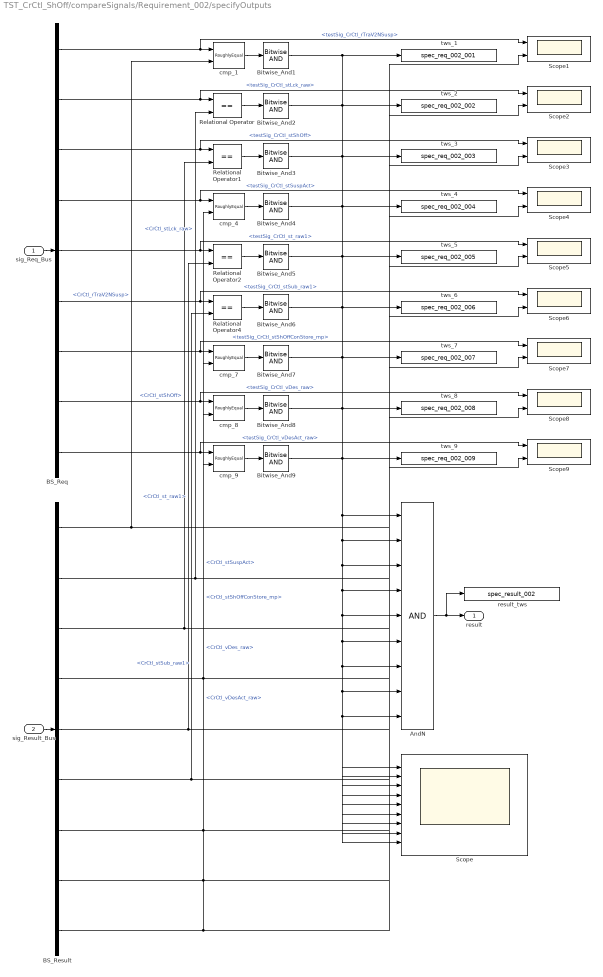
== system TST_CrCtl_ShOff/compareSignals/Requirement_002/specifyOutputs ==
  sig_Req_Bus : Inport
  sig_Result_Bus : Inport  Port=2
  AndN : Logic  Inputs=9
  BS_Req : BusSelector  OutputSignals=testSig_CrCtl_rTraV2NSusp,testSig_CrCtl_stLck_raw,testSig_CrCtl_stShOff,testSig_CrCtl_stSuspAct,testSig_CrCtl_st_raw1,testSig_CrCtl_stSub_raw1,testSig_CrCtl_stShOffConStore_mp,testSig_CrCtl_vDes_raw,testSig_CrCtl_vDesAct_raw
  BS_Result : BusSelector  OutputSignals=CrCtl_rTraV2NSusp,CrCtl_stLck_raw,CrCtl_stShOff,CrCtl_stSuspAct,CrCtl_st_raw1,CrCtl_stSub_raw1,CrCtl_stShOffConStore_mp,CrCtl_vDes_raw,CrCtl_vDesAct_raw
  Bitwise_And{1..9} (9 alike) : simulink/Logic and Bit Operations/Bitwise Operator  logicop=AND  UseBitMask=off  BitMask=bin2dec('11011001')  BitMaskRealWorld=Stored Integer
  Relational Operator{,1..2,4} (4 alike) : RelationalOperator  Operator===  OutDataTypeStr=boolean  RndMeth=Simplest
  Scope : Scope  NumInputPorts=9
  Scope{1..9} (9 alike) : Scope  NumInputPorts=2
  cmp_{1,4,7..9} (5 alike) : UnitTest_Lib/RoughlyEqual  slope=0.1
  result_tws : ToWorkspace  VariableName=spec_result_002
  tws_1 : ToWorkspace  VariableName=spec_req_002_001
  tws_2 : ToWorkspace  VariableName=spec_req_002_002
  tws_3 : ToWorkspace  VariableName=spec_req_002_003
  tws_4 : ToWorkspace  VariableName=spec_req_002_004
  tws_5 : ToWorkspace  VariableName=spec_req_002_005
  tws_6 : ToWorkspace  VariableName=spec_req_002_006
  tws_7 : ToWorkspace  VariableName=spec_req_002_007
  tws_8 : ToWorkspace  VariableName=spec_req_002_008
  tws_9 : ToWorkspace  VariableName=spec_req_002_009
  result : Outport
  wires:
  sig_Req_Bus/1 -> BS_Req/1
  sig_Result_Bus/1 -> BS_Result/1
  AndN/1 -> result/1, result_tws/1
  BS_Req/1 -> cmp_1/1, Scope1/1  "<testSig_CrCtl_rTraV2NSusp>"
  BS_Result/1 -> cmp_1/2, Scope1/2  "<CrCtl_rTraV2NSusp>"
  cmp_1/1 -> Bitwise_And1/1
  Bitwise_And1/1 -> AndN/1, Scope/1, tws_1/1
  BS_Req/2 -> Relational Operator/1, Scope2/1  "<testSig_CrCtl_stLck_raw>"
  BS_Result/2 -> Scope2/2, Relational Operator/2  "<CrCtl_stLck_raw>"
  Relational Operator/1 -> Bitwise_And2/1
  Bitwise_And2/1 -> AndN/2, Scope/2, tws_2/1
  BS_Req/3 -> Relational Operator1/1, Scope3/1  "<testSig_CrCtl_stShOff>"
  BS_Result/3 -> Scope3/2, Relational Operator1/2  "<CrCtl_stShOff>"
  Relational Operator1/1 -> Bitwise_And3/1
  Bitwise_And3/1 -> AndN/3, Scope/3, tws_3/1
  BS_Req/4 -> cmp_4/1, Scope4/1  "<testSig_CrCtl_stSuspAct>"
  BS_Result/4 -> cmp_4/2, Scope4/2  "<CrCtl_stSuspAct>"
  cmp_4/1 -> Bitwise_And4/1
  Bitwise_And4/1 -> AndN/4, Scope/4, tws_4/1
  BS_Req/5 -> Relational Operator2/1, Scope5/1  "<testSig_CrCtl_st_raw1>"
  BS_Result/5 -> Scope5/2, Relational Operator2/2  "<CrCtl_st_raw1>"
  Relational Operator2/1 -> Bitwise_And5/1
  Bitwise_And5/1 -> AndN/5, Scope/5, tws_5/1
  BS_Req/6 -> Relational Operator4/1, Scope6/1  "<testSig_CrCtl_stSub_raw1>"
  BS_Result/6 -> Scope6/2, Relational Operator4/2  "<CrCtl_stSub_raw1>"
  Relational Operator4/1 -> Bitwise_And6/1
  Bitwise_And6/1 -> AndN/6, Scope/6, tws_6/1
  BS_Req/7 -> cmp_7/1, Scope7/1  "<testSig_CrCtl_stShOffConStore_mp>"
  BS_Result/7 -> cmp_7/2, Scope7/2  "<CrCtl_stShOffConStore_mp>"
  cmp_7/1 -> Bitwise_And7/1
  Bitwise_And7/1 -> AndN/7, Scope/7, tws_7/1
  BS_Req/8 -> cmp_8/1, Scope8/1  "<testSig_CrCtl_vDes_raw>"
  BS_Result/8 -> cmp_8/2, Scope8/2  "<CrCtl_vDes_raw>"
  cmp_8/1 -> Bitwise_And8/1
  Bitwise_And8/1 -> AndN/8, Scope/8, tws_8/1
  BS_Req/9 -> cmp_9/1, Scope9/1  "<testSig_CrCtl_vDesAct_raw>"
  BS_Result/9 -> cmp_9/2, Scope9/2  "<CrCtl_vDesAct_raw>"
  cmp_9/1 -> Bitwise_And9/1
  Bitwise_And9/1 -> AndN/9, Scope/9, tws_9/1

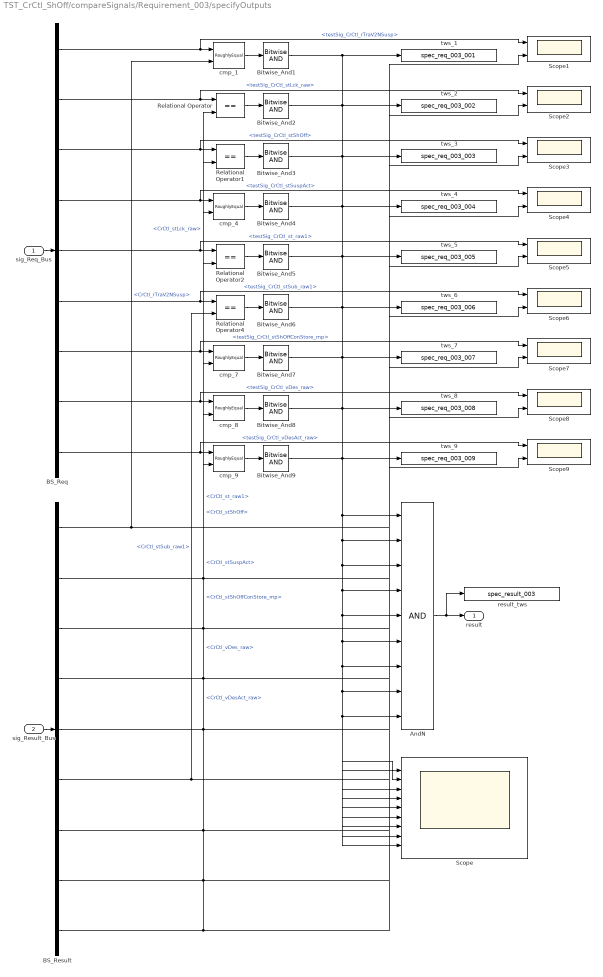
== system TST_CrCtl_ShOff/compareSignals/Requirement_003/specifyOutputs ==
  sig_Req_Bus : Inport
  sig_Result_Bus : Inport  Port=2
  AndN : Logic  Inputs=9
  BS_Req : BusSelector  OutputSignals=testSig_CrCtl_rTraV2NSusp,testSig_CrCtl_stLck_raw,testSig_CrCtl_stShOff,testSig_CrCtl_stSuspAct,testSig_CrCtl_st_raw1,testSig_CrCtl_stSub_raw1,testSig_CrCtl_stShOffConStore_mp,testSig_CrCtl_vDes_raw,testSig_CrCtl_vDesAct_raw
  BS_Result : BusSelector  OutputSignals=CrCtl_rTraV2NSusp,CrCtl_stLck_raw,CrCtl_stShOff,CrCtl_stSuspAct,CrCtl_st_raw1,CrCtl_stSub_raw1,CrCtl_stShOffConStore_mp,CrCtl_vDes_raw,CrCtl_vDesAct_raw
  Bitwise_And{1..9} (9 alike) : simulink/Logic and Bit Operations/Bitwise Operator  logicop=AND  UseBitMask=off  BitMask=bin2dec('11011001')  BitMaskRealWorld=Stored Integer
  Relational Operator{,1..2,4} (4 alike) : RelationalOperator  Operator===  OutDataTypeStr=boolean  RndMeth=Simplest
  Scope : Scope  NumInputPorts=9
  Scope{1..9} (9 alike) : Scope  NumInputPorts=2
  cmp_{1,4,7..9} (5 alike) : UnitTest_Lib/RoughlyEqual  slope=0.1
  result_tws : ToWorkspace  VariableName=spec_result_003
  tws_1 : ToWorkspace  VariableName=spec_req_003_001
  tws_2 : ToWorkspace  VariableName=spec_req_003_002
  tws_3 : ToWorkspace  VariableName=spec_req_003_003
  tws_4 : ToWorkspace  VariableName=spec_req_003_004
  tws_5 : ToWorkspace  VariableName=spec_req_003_005
  tws_6 : ToWorkspace  VariableName=spec_req_003_006
  tws_7 : ToWorkspace  VariableName=spec_req_003_007
  tws_8 : ToWorkspace  VariableName=spec_req_003_008
  tws_9 : ToWorkspace  VariableName=spec_req_003_009
  result : Outport
  wires:
  sig_Req_Bus/1 -> BS_Req/1
  sig_Result_Bus/1 -> BS_Result/1
  AndN/1 -> result/1, result_tws/1
  BS_Req/1 -> cmp_1/1, Scope1/1  "<testSig_CrCtl_rTraV2NSusp>"
  BS_Result/1 -> cmp_1/2, Scope1/2  "<CrCtl_rTraV2NSusp>"
  cmp_1/1 -> Bitwise_And1/1
  Bitwise_And1/1 -> AndN/1, Scope/1, tws_1/1
  BS_Req/2 -> Relational Operator/1, Scope2/1  "<testSig_CrCtl_stLck_raw>"
  BS_Result/2 -> Relational Operator/2, Scope2/2  "<CrCtl_stLck_raw>"
  Relational Operator/1 -> Bitwise_And2/1
  Bitwise_And2/1 -> AndN/2, Scope/2, tws_2/1
  BS_Req/3 -> Relational Operator1/1, Scope3/1  "<testSig_CrCtl_stShOff>"
  BS_Result/3 -> Relational Operator1/2, Scope3/2  "<CrCtl_stShOff>"
  Relational Operator1/1 -> Bitwise_And3/1
  Bitwise_And3/1 -> AndN/3, Scope/3, tws_3/1
  BS_Req/4 -> cmp_4/1, Scope4/1  "<testSig_CrCtl_stSuspAct>"
  BS_Result/4 -> cmp_4/2, Scope4/2  "<CrCtl_stSuspAct>"
  cmp_4/1 -> Bitwise_And4/1
  Bitwise_And4/1 -> AndN/4, Scope/4, tws_4/1
  BS_Req/5 -> Relational Operator2/1, Scope5/1  "<testSig_CrCtl_st_raw1>"
  BS_Result/5 -> Relational Operator2/2, Scope5/2  "<CrCtl_st_raw1>"
  Relational Operator2/1 -> Bitwise_And5/1
  Bitwise_And5/1 -> AndN/5, Scope/5, tws_5/1
  BS_Req/6 -> Relational Operator4/1, Scope6/1  "<testSig_CrCtl_stSub_raw1>"
  BS_Result/6 -> Scope6/2, Relational Operator4/2  "<CrCtl_stSub_raw1>"
  Relational Operator4/1 -> Bitwise_And6/1
  Bitwise_And6/1 -> AndN/6, Scope/6, tws_6/1
  BS_Req/7 -> cmp_7/1, Scope7/1  "<testSig_CrCtl_stShOffConStore_mp>"
  BS_Result/7 -> cmp_7/2, Scope7/2  "<CrCtl_stShOffConStore_mp>"
  cmp_7/1 -> Bitwise_And7/1
  Bitwise_And7/1 -> AndN/7, Scope/7, tws_7/1
  BS_Req/8 -> cmp_8/1, Scope8/1  "<testSig_CrCtl_vDes_raw>"
  BS_Result/8 -> cmp_8/2, Scope8/2  "<CrCtl_vDes_raw>"
  cmp_8/1 -> Bitwise_And8/1
  Bitwise_And8/1 -> AndN/8, Scope/8, tws_8/1
  BS_Req/9 -> cmp_9/1, Scope9/1  "<testSig_CrCtl_vDesAct_raw>"
  BS_Result/9 -> cmp_9/2, Scope9/2  "<CrCtl_vDesAct_raw>"
  cmp_9/1 -> Bitwise_And9/1
  Bitwise_And9/1 -> AndN/9, Scope/9, tws_9/1
